simulink model "merge_test"  (Simulink 8.4)
settings: Solver=VariableStepDiscrete  StartTime=0.0  StopTime=0  MaxStep=1  RelTol=1e-3
settings Model: Creator=arnaud  LastModifiedBy=arnaud
settings DataIOCC: ExternalInput=xin  SaveFormat=Structure

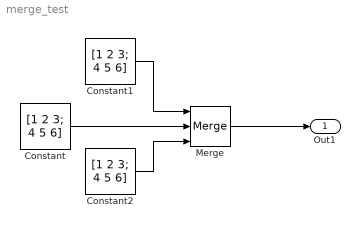
== system merge_test ==
  Constant : Constant  Value=[1 2 3; 4 5 6]
  Constant1 : Constant  Value=[1 2 3; 4 5 6]
  Constant2 : Constant  Value=[1 2 3; 4 5 6]
  Merge : Merge  Inputs=3
  Out1 : Outport
  wires:
  Merge/1 -> Out1/1
  Constant1/1 -> Merge/1
  Constant/1 -> Merge/2
  Constant2/1 -> Merge/3
